simulink model "Gercek_Model_Non_Linear_Ters_Sarkac"  (R2022a)
settings: Solver=ode4  StartTime=0.0  StopTime=20  FixedStep=1/1000  RelTol=1e-3
InitFcn:
  | Sarkac_Parametrelerini_Yukle
values from neighbouring files (symbols this model uses):
  b = 0.1    [Sarkac_Parametrelerini_Yukle.m]
  Baslangic_Degerleri = [0,0,pi,0]    [Sarkac_Parametrelerini_Yukle.m]
  g = 9.8    [Sarkac_Parametrelerini_Yukle.m]
  I = 0.006    [Sarkac_Parametrelerini_Yukle.m]
  l = 0.3    [Sarkac_Parametrelerini_Yukle.m]
  LQR_Katsayi_Matrisi = [-9.9999999999999627 -18.743235127431934 128.16450584818944                         40.177837789932831]    [Sarkac_Parametrelerini_Yukle.m]
  M = 0.5    [Sarkac_Parametrelerini_Yukle.m]
  m = 0.2    [Sarkac_Parametrelerini_Yukle.m]
libraries: simulink_extras x2, vrlib x1
settings Model: Creator=Fatabi  LastModifiedBy=Fatabi
settings SolverCC: AlgebraicLoopSolver=TrustRegion
settings DebuggingCC: UnconnectedInputMsg=warning  UnconnectedOutputMsg=warning  UnconnectedLineMsg=warning  SFMachineParentedDataDiag=warning

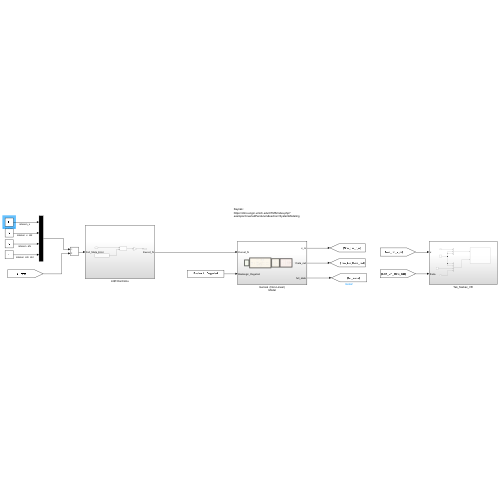
[thumbnail: Simulink's stored preview of the top-level diagram]
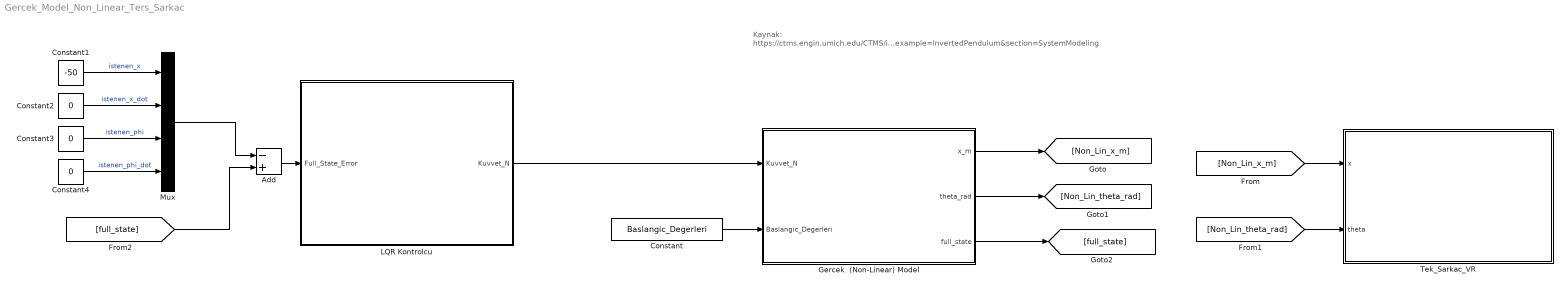
== system Gercek_Model_Non_Linear_Ters_Sarkac ==
  note: Kaynak:
      | https://ctms.engin.umich.edu/CTMS/index.php?example=InvertedPendulum&section=SystemModeling
  Add : Sum  Inputs=-+
  Constant : Constant  Value=Baslangic_Degerleri
  Constant1 : Constant  Value=-50
  Constant2 : Constant  Value=0
  Constant3 : Constant  Value=0
  Constant4 : Constant  Value=0
  Gercek  (Non-Linear) Model : Subsystem
  LQR Kontrolcu : Subsystem
  Mux : Mux
  "Tek_Sarkac_VR " : Subsystem
  wires:
  LQR Kontrolcu/1(Kuvvet_N) -> Gercek  (Non-Linear) Model/1(Kuvvet_N)
  Constant/1 -> Gercek  (Non-Linear) Model/2(Baslangic_Degerleri)
  Gercek  (Non-Linear) Model/1(x_m) -> [Non_Lin_x_m]
  Gercek  (Non-Linear) Model/2(theta_rad) -> [Non_Lin_theta_rad]
  [Non_Lin_x_m] -> "Tek_Sarkac_VR "/1(x)
  [Non_Lin_theta_rad] -> "Tek_Sarkac_VR "/2("theta ")
  Add/1 -> LQR Kontrolcu/1(Full_State_Error)
  Mux/1 -> Add/1
  Constant4/1 -> Mux/4  "istenen_phi_dot"
  Constant3/1 -> Mux/3  "istenen_phi"
  Constant1/1 -> Mux/1  "istenen_x"
  Constant2/1 -> Mux/2  "istenen_x_dot"
  [full_state] -> Add/2
  Gercek  (Non-Linear) Model/3(full_state) -> [full_state]

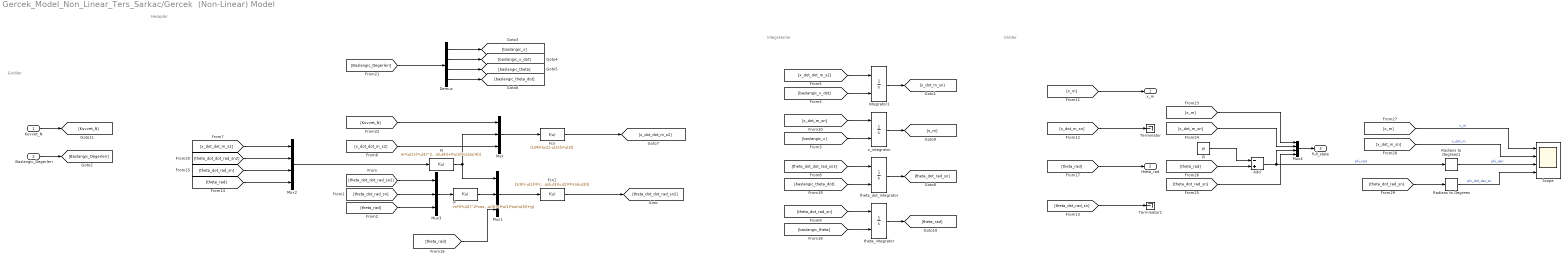
== system Gercek_Model_Non_Linear_Ters_Sarkac/Gercek  (Non-Linear) Model ==
  note: Integratorler
  note: Girdiler
  note: Ciktilar
  note: Hesaplar
  Kuvvet_N : Inport
  Baslangic_Degerleri : Inport  Port=2
  Add : Sum  Inputs=-+
  Demux : Demux
  Fcn : Fcn  Expr=(1/M)*(u(1)-u(2)-b*u(3))
  Fcn1 : Fcn  Expr=(1/I)*(-u(1)*l*cos(u(3))-u(2)*l*sin(u(3)))
  Integrator1 : Integrator  InitialConditionSource=external  ContinuousStateAttributes='x_dot_m_sn'
  Mux : Mux  Inputs=3
  Mux1 : Mux  Inputs=3
  Mux2 : Mux
  Mux3 : Mux  Inputs=3
  Mux4 : Mux
  N : Fcn  Expr=m*(u(1)-l*u(3)^2*sin(u(4))+l*u(2)*cos(u(4)))
  P : Fcn  Expr=m*(l*u(2)^2*cos(u(3))+l*u(1)*sin(u(3))+g)
  Pi : Constant  Value=pi  OutDataTypeStr=Inherit: Inherit via back propagation
  Radians to Degrees : simulink_extras/Transformations/Radians to Degrees
  Radians to Degrees1 : simulink_extras/Transformations/Radians to Degrees
  Scope : Scope  NumInputPorts=4
  Terminator : Terminator
  Terminator1 : Terminator
  theta_dot_integrator : Integrator  InitialConditionSource=external  ContinuousStateAttributes='theta_dot_rad_sn'
  theta_integrator : Integrator  InitialConditionSource=external  InitialCondition=pi-0.1  ContinuousStateAttributes='theta_rad'
  x_integrator : Integrator  InitialConditionSource=external  ContinuousStateAttributes='x_m'
  x_m : Outport
  theta_rad : Outport  Port=2
  full_state : Outport  Port=3
  wires:
  [x_dot_dot_m_s2] -> Mux/3
  Fcn/1 -> [x_dot_dot_m_s2]
  [Kuvvet_N] -> Mux/1
  N/1 -> Mux1/1, Mux/2
  Mux/1 -> Fcn/1
  Fcn1/1 -> [theta_dot_dot_rad_sn2]
  Mux1/1 -> Fcn1/1
  P/1 -> Mux1/2
  Mux2/1 -> N/1
  [theta_dot_dot_rad_sn2] -> Mux3/1
  [theta_dot_rad_sn] -> Mux3/2
  [theta_rad] -> Mux3/3
  Mux3/1 -> P/1
  [Baslangic_Degerleri] -> Demux/1
  Demux/1 -> [baslangic_x]
  Demux/2 -> [baslangic_x_dot]
  Demux/3 -> [baslangic_theta]
  Demux/4 -> [baslangic_theta_dot]
  [baslangic_x] -> x_integrator/2
  x_integrator/1 -> [x_m]
  [baslangic_x_dot] -> Integrator1/2
  [x_dot_dot_m_s2] -> Integrator1/1
  Integrator1/1 -> [x_dot_m_sn]
  [x_dot_dot_m_s2] -> Mux2/1
  [theta_dot_dot_rad_sn2] -> theta_dot_integrator/1
  theta_dot_integrator/1 -> [theta_dot_rad_sn]
  [x_dot_m_sn] -> x_integrator/1
  [x_m] -> x_m/1
  [x_dot_m_sn] -> Terminator/1
  [theta_dot_rad_sn] -> theta_integrator/1
  theta_integrator/1 -> [theta_rad]
  [theta_rad] -> Mux2/4
  [theta_dot_rad_sn] -> Mux2/3
  [theta_rad] -> Mux1/3
  [theta_rad] -> theta_rad/1
  [baslangic_theta] -> theta_integrator/2
  [baslangic_theta_dot] -> theta_dot_integrator/2
  [theta_dot_dot_rad_sn2] -> Mux2/2
  Baslangic_Degerleri/1 -> [Baslangic_Degerleri]
  Kuvvet_N/1 -> [Kuvvet_N]
  [theta_dot_rad_sn] -> Terminator1/1
  [theta_rad] -> Add/2
  Pi/1 -> Add/1
  Add/1 -> Mux4/3, Radians to Degrees1/1  "phi_rad"
  [x_dot_m_sn] -> Mux4/2
  [theta_dot_rad_sn] -> Mux4/4
  [x_m] -> Mux4/1
  Mux4/1 -> full_state/1
  Radians to Degrees/1 -> Scope/4  "phi_dot_der_sn"
  [x_dot_m_sn] -> Scope/2  "x_dot_m"
  [x_m] -> Scope/1  "x_m"
  Radians to Degrees1/1 -> Scope/3  "phi_der"
  [theta_dot_rad_sn] -> Radians to Degrees/1

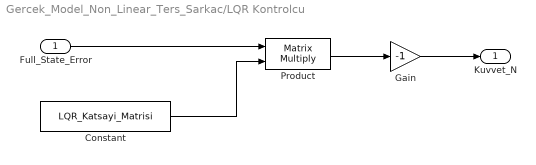
== system Gercek_Model_Non_Linear_Ters_Sarkac/LQR Kontrolcu ==
  Full_State_Error : Inport
  Constant : Constant  Value=LQR_Katsayi_Matrisi
  Gain : Gain  Gain=-1
  Product : Product  Multiplication=Matrix(*)
  Kuvvet_N : Outport
  wires:
  Gain/1 -> Kuvvet_N/1
  Product/1 -> Gain/1
  Full_State_Error/1 -> Product/1
  Constant/1 -> Product/2

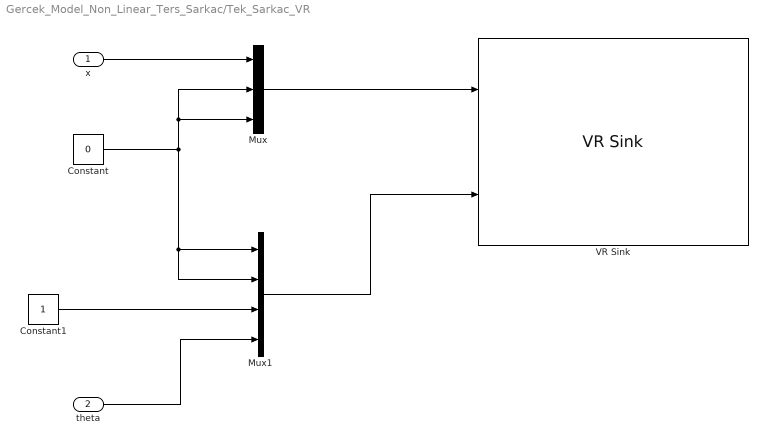
== system Gercek_Model_Non_Linear_Ters_Sarkac/Tek_Sarkac_VR  ==
  x : Inport
  "theta " : Inport  Port=2
  Constant : Constant  Value=0
  Constant1 : Constant
  Mux : Mux  Inputs=3
  Mux1 : Mux
  VR Sink : vrlib/VR Sink  InstantiateOnLoad=on  SampleTime=0.02  ViewEnable=on  RemoteChange=off  RemoteView=off  FieldsWritten=Kutu.translation.3.1.1.double#Mentese1.rotation.4.1.1.double  WorldFileName=sarkac.wrl  AutoView=off  VideoDimensions=[]  AllowVariableSize=off
  wires:
  x/1 -> Mux/1
  Constant/1 -> Mux/3, Mux/2, Mux1/2, Mux1/1
  "theta "/1 -> Mux1/4
  Constant1/1 -> Mux1/3
  Mux/1 -> VR Sink/1
  Mux1/1 -> VR Sink/2
